simulink model "PMSM_control_model"  (R2024b)
settings: Solver=VariableStepAuto  StartTime=0.0  StopTime=3  RelTol=1e-3
values from neighbouring files (symbols this model uses):
  Is_max = 16    [PMSM_control.m]
  Ls = 5.5e-3    (= 0.0055)    [PMSM_control.m]
  Lsd = 5.5e-3    (= 0.0055)    [PMSM_control.m]
  p = 2    [PMSM_control.m]
  psi_f = 75e-3    (= 0.075)    [PMSM_control.m]
  Us_max = 60    [PMSM_control.m]
libraries: mcbcontrolslib x5, simulink x2
settings Model: Creator=chinm  LastModifiedBy=chinm

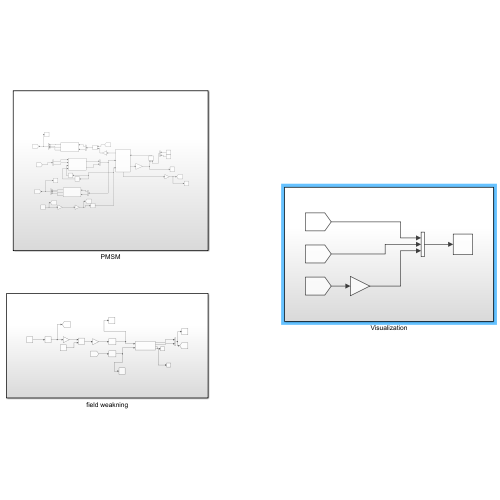
[thumbnail: Simulink's stored preview of the top-level diagram]
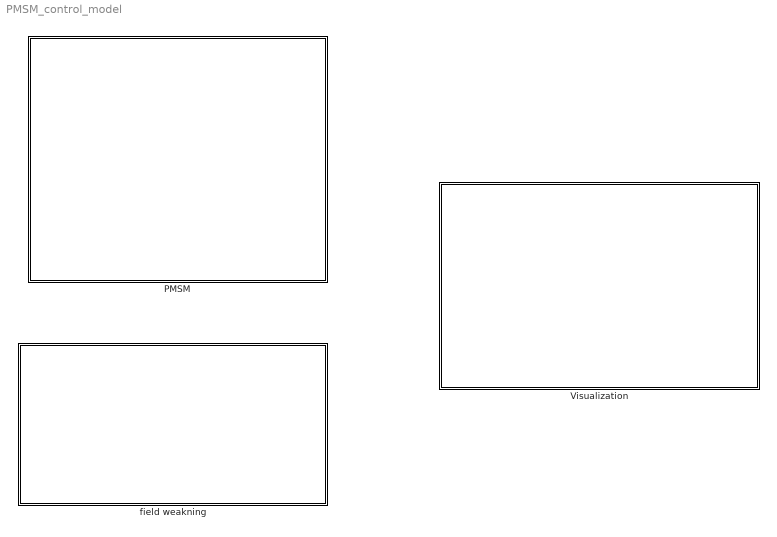
== system PMSM_control_model ==
  PMSM : Subsystem
  Visualization : Subsystem
  field weakning : Subsystem

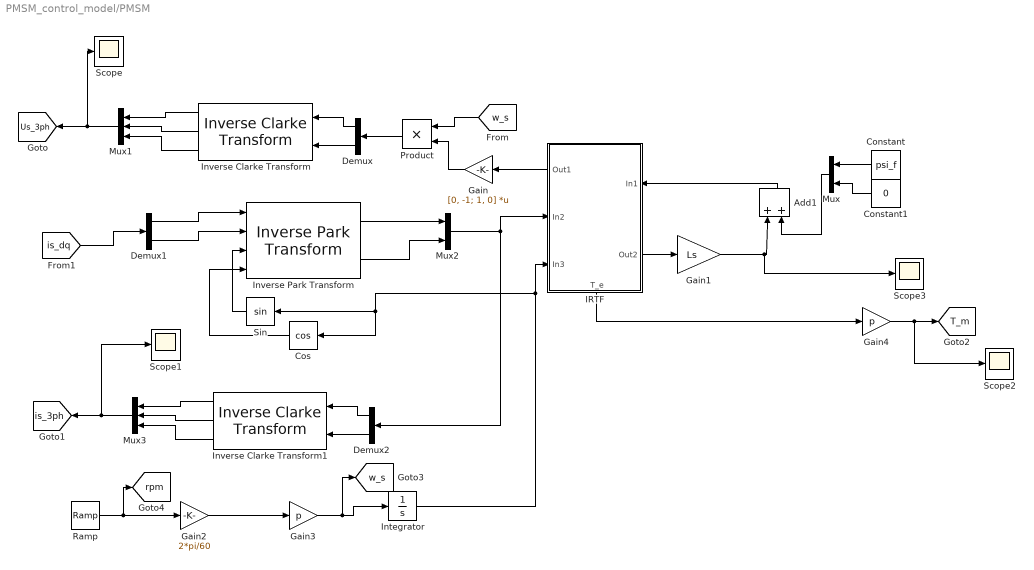
== system PMSM_control_model/PMSM ==
  Add1 : Sum
  Constant : Constant  Value=psi_f
  Constant1 : Constant  Value=0
  Cos : Trigonometry  Operator=cos
  Demux : Demux  Outputs=2
  Demux1 : Demux  Outputs=2
  Demux2 : Demux  Outputs=2
  Gain : Gain  Gain=[0, -1; 1, 0]  Multiplication=Matrix(K*u)
  Gain1 : Gain  Gain=Ls
  Gain2 : Gain  Gain=2*pi/60
  Gain3 : Gain  Gain=p
  Gain4 : Gain  Gain=p
  IRTF : Subsystem
      settings: PortSchema="{\"entries\":[{\"content\":{\"sides\":[{\"content\":{\"connectorIds\":[\"Out3\",\"In1\",\"In2\"]},\"type\":\"ConnectorPlacement.EquallySpacedRectSide\",\"uuid\":\"b4986fb2-c57d-4b73-a735-292653fff6d9\"},{\"content\":{\"connectorIds\":[\"In3\",\"Out1\"],\"side\":\"RIGHT\"},\"type\":\"ConnectorPlacement.EquallySpacedRectSide\",\"uuid\":\"9d0dc8a9-3fda-4760-870c-c4cad97d429b\"},{\"content\":{\"side\":\"TOP\"},\"type\":\"ConnectorPlacement.EquallySpacedRectSide\",\"uuid\":\"e1f646a3-730d-45a9-a867-cd53dcd150be\"},{\"content\":{\"connectorIds\":[\"Out2\"],\"side\":\"BOTTOM\"},\"type\":\"ConnectorPlacement.EquallySpacedRectSide\",\"uuid\":\"c6f4b204-5ea6-4623-acea-3e4f968e6d8a\"}]},\"type\":\"ConnectorPlacement.EquallySpacedConnector\",\"uuid\":\"ab7f54df-393a-4b01-99b4-3432e63bf963\"}],\"packageUris\":[\"http://schema.mathworks.com/mf0/Connector/R2020b\"],\"version\":\"1.0\"}"
  Integrator : Integrator
  Inverse Clarke Transform : mcbcontrolslib/Inverse Clarke Transform  PhaseInput=Two inputs  EnPowerInv=off
      settings: LibrarySourceBlock=mcblib/Controls/Math Transforms/Inverse Clarke Transform
  Inverse Clarke Transform1 : mcbcontrolslib/Inverse Clarke Transform  PhaseInput=Two inputs  EnPowerInv=off
      settings: LibrarySourceBlock=mcblib/Controls/Math Transforms/Inverse Clarke Transform
  Inverse Park Transform : mcbcontrolslib/Inverse Park Transform  PhaseInput=Two inputs  AxisAlignment=D-axis  ThetaInput=Sine and Cosine electrical position  AngleInput=Per-unit  N_points=1024
      settings: LibrarySourceBlock=mcbhdllib/Controls/Math Transforms/Inverse Park Transform
  Mux : Mux  Inputs=2
  Mux1 : Mux  Inputs=3
  Mux2 : Mux  Inputs=2
  Mux3 : Mux  Inputs=3
  Product : Product
  Ramp : simulink/Sources/Ramp  slope=5000  start=0  InitialOutput=0
  Scope{,1..3} (4 alike) : Scope
  Sin : Trigonometry
  tag scope: T_m=global, Us_3ph=global, is_3ph=global, rpm=global, w_s=global
  wires:
  Constant/1 -> Mux/1
  Constant1/1 -> Mux/2
  Mux/1 -> Add1/2
  Integrator/1 -> IRTF/2(In3), Cos/1, Sin/1
  IRTF/2(T_e) -> Gain4/1
  IRTF/1(Out2) -> Gain1/1
  Gain1/1 -> Scope3/1, Add1/1
  Add1/1 -> IRTF/3(In1)
  IRTF/3(Out1) -> Gain/1
  Gain/1 -> Product/2
  [w_s] -> Product/1
  Product/1 -> Demux/1
  Demux/1 -> Inverse Clarke Transform/1
  Demux/2 -> Inverse Clarke Transform/2
  Mux1/1 -> Scope/1, [Us_3ph]
  Inverse Clarke Transform/1 -> Mux1/1
  Inverse Clarke Transform/2 -> Mux1/2
  Inverse Clarke Transform/3 -> Mux1/3
  Inverse Park Transform/1 -> Mux2/1
  Inverse Park Transform/2 -> Mux2/2
  Sin/1 -> Inverse Park Transform/3
  Cos/1 -> Inverse Park Transform/4
  Demux1/1 -> Inverse Park Transform/1
  Demux1/2 -> Inverse Park Transform/2
  [is_dq] -> Demux1/1
  Demux2/2 -> Inverse Clarke Transform1/2
  Inverse Clarke Transform1/3 -> Mux3/3
  Inverse Clarke Transform1/2 -> Mux3/2
  Inverse Clarke Transform1/1 -> Mux3/1
  Mux2/1 -> IRTF/1(In2), Demux2/1
  Mux3/1 -> Scope1/1, [is_3ph]
  Demux2/1 -> Inverse Clarke Transform1/1
  Gain2/1 -> Gain3/1
  Gain3/1 -> [w_s], Integrator/1
  Gain4/1 -> Scope2/1, [T_m]
  Ramp/1 -> [rpm], Gain2/1

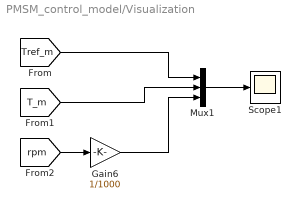
== system PMSM_control_model/Visualization ==
  Gain6 : Gain  Gain=1/1000
  Mux1 : Mux  Inputs=3
  Scope1 : Scope
  wires:
  Mux1/1 -> Scope1/1
  [T_m] -> Mux1/2
  [rpm] -> Gain6/1
  Gain6/1 -> Mux1/3
  [Tref_m] -> Mux1/1

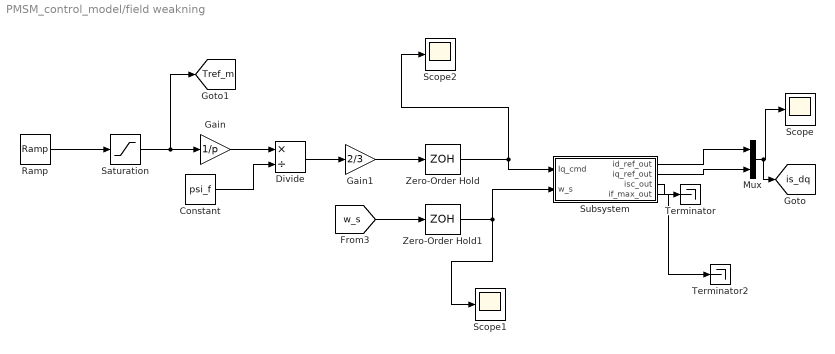
== system PMSM_control_model/field weakning ==
  Constant : Constant  Value=psi_f
  Divide : Product  Inputs=*/
  Gain : Gain  Gain=1/p
  Gain1 : Gain  Gain=2/3
  Mux : Mux  Inputs=2
  Ramp : simulink/Sources/Ramp  slope=10  start=0  InitialOutput=0
  Saturation : Saturate  UpperLimit=2  LowerLimit=0
  Scope : Scope
  Scope1 : Scope
  Scope2 : Scope
  Subsystem : Subsystem
  Terminator : Terminator
  Terminator2 : Terminator
  Zero-Order Hold : ZeroOrderHold  SampleTime=1e-4
  Zero-Order Hold1 : ZeroOrderHold  SampleTime=1e-4
  tag scope: Tref_m=global, is_dq=global
  wires:
  Zero-Order Hold1/1 -> Scope1/1, Subsystem/2(w_s)
  Constant/1 -> Divide/2
  Saturation/1 -> [Tref_m], Gain/1
  Mux/1 -> [is_dq], Scope/1
  Gain/1 -> Divide/1
  [w_s] -> Zero-Order Hold1/1
  Gain1/1 -> Zero-Order Hold/1
  Zero-Order Hold/1 -> Scope2/1, Subsystem/1(Iq_cmd)
  Divide/1 -> Gain1/1
  Subsystem/1(id_ref_out) -> Mux/1
  Subsystem/2(iq_ref_out) -> Mux/2
  Subsystem/3(isc_out) -> Terminator/1
  Subsystem/4(if_max_out) -> Terminator2/1
  Ramp/1 -> Saturation/1

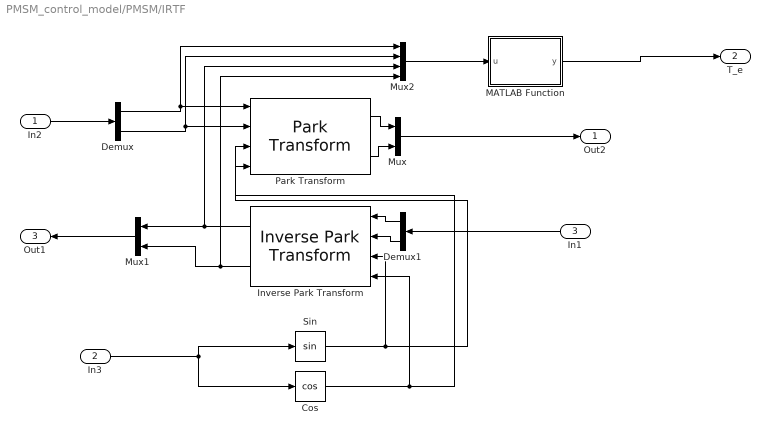
== system PMSM_control_model/PMSM/IRTF ==
  In2 : Inport
  In3 : Inport  Port=2
  In1 : Inport  Port=3
  Cos : Trigonometry  Operator=cos
  Demux : Demux  Outputs=2
  Demux1 : Demux  Outputs=2
  Inverse Park Transform : mcbcontrolslib/Inverse Park Transform  PhaseInput=Two inputs  AxisAlignment=D-axis  ThetaInput=Sine and Cosine electrical position  AngleInput=Per-unit  N_points=1024
  MATLAB Function : MATLAB Function  TreatAsAtomicUnit=on
  Mux : Mux  Inputs=2
  Mux1 : Mux  Inputs=2
  Mux2 : Mux
  Park Transform : mcbcontrolslib/Park Transform  PhaseInput=Two inputs  AxisAlignment=D-axis  ThetaInput=Sine and Cosine electrical position  AngleInput=Per-unit  N_points=1024
  Sin : Trigonometry
  Out2 : Outport
  T_e : Outport  Port=2
  Out1 : Outport  Port=3
  wires:
  Demux/1 -> Mux2/1, Park Transform/1
  Demux/2 -> Mux2/2, Park Transform/2
  Park Transform/1 -> Mux/1
  Park Transform/2 -> Mux/2
  Demux1/1 -> Inverse Park Transform/1
  Demux1/2 -> Inverse Park Transform/2
  Inverse Park Transform/1 -> Mux2/3, Mux1/1
  Inverse Park Transform/2 -> Mux2/4, Mux1/2
  In3/1 -> Sin/1, Cos/1
  Sin/1 -> Park Transform/3, Inverse Park Transform/3
  Cos/1 -> Park Transform/4, Inverse Park Transform/4
  Mux2/1 -> MATLAB Function/1(u)
  MATLAB Function/1(y) -> T_e/1
  In1/1 -> Demux1/1
  Mux1/1 -> Out1/1
  In2/1 -> Demux/1
  Mux/1 -> Out2/1

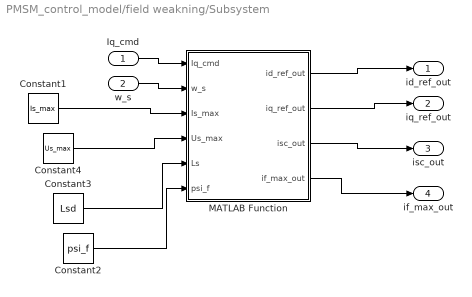
== system PMSM_control_model/field weakning/Subsystem ==
  Iq_cmd : Inport
  w_s : Inport  Port=2
  Constant1 : Constant  Value=Is_max
  Constant2 : Constant  Value=psi_f
  Constant3 : Constant  Value=Lsd
  Constant4 : Constant  Value=Us_max
  MATLAB Function : MATLAB Function  TreatAsAtomicUnit=on
  id_ref_out : Outport
  iq_ref_out : Outport  Port=2
  isc_out : Outport  Port=3
  if_max_out : Outport  Port=4
  wires:
  MATLAB Function/1(id_ref_out) -> id_ref_out/1
  MATLAB Function/2(iq_ref_out) -> iq_ref_out/1
  MATLAB Function/3(isc_out) -> isc_out/1
  MATLAB Function/4(if_max_out) -> if_max_out/1
  Iq_cmd/1 -> MATLAB Function/1(Iq_cmd)
  w_s/1 -> MATLAB Function/2(w_s)
  Constant1/1 -> MATLAB Function/3(Is_max)
  Constant2/1 -> MATLAB Function/6(psi_f)
  Constant3/1 -> MATLAB Function/5(Ls)
  Constant4/1 -> MATLAB Function/4(Us_max)

== matlab function PMSM_control_model/field weakning/Subsystem/MATLAB Function ==
  data: Iq_cmd input; id_ref_out output; w_s input; Is_max input; Us_max input; Ls input; psi_f input; iq_ref_out output; isc_out output; if_max_out output
function [id_ref_out, iq_ref_out, isc_out, if_max_out] = control_logic(Iq_cmd, w_s, Is_max, Us_max, Ls, psi_f)
    % Avoid division by zero
    w_s = max(abs(w_s), 1e-3);
    current = abs(Iq_cmd);

    % Limit current to Is_max
    if current > Is_max
        current = Is_max;
    end

    % Base quantities
    iflm = Us_max / (w_s * Ls);  % voltage ellipse radius
    isc = psi_f / Ls;            % short-circuit current

    % Intersection of voltage ellipse with iq-axis (id = 0)
    iflmq = 0;
    if isc < iflm
        iflmq = sqrt(iflm^2 - isc^2);
    end

    % === Case 1: MTPA ===
    id_ref_MTPA = 0;
    iq_ref_MTPA = current;

    % === Case 2: Field Weakening ===
    iq_ref_FW = current;
    if iflm < current
        iq_ref_FW = iflm;
    end
    temp_fw = max(0, iflm^2 - iq_ref_FW^2);
    id_ref_FW = sqrt(temp_fw) - isc;

    % === Case 3: Maximum Acceleration (MA) ===
    id_ref_MA = (iflm^2 - Is_max^2 - isc^2) / (2 * isc);
    iq_ref_MA = sqrt(max(0, Is_max^2 - id_ref_MA^2));

    % === Default: MTPA ===
    id_ref = id_ref_MTPA;
    iq_ref = iq_ref_MTPA;

    % === FW Mode Trigger ===
    if iq_ref_MTPA > iflmq
        id_ref = id_ref_FW;
        iq_ref = iq_ref_FW;
    end

    % === MA Mode Trigger ===
    if (id_ref^2 + iq_ref^2) > Is_max^2
        id_ref = id_ref_MA;
        iq_ref = iq_ref_MA;
    end

    % === Final Outputs ===
    id_ref_out = id_ref;
    iq_ref_out = iq_ref;
    isc_out = isc;
    if_max_out = iflm;
end

== matlab function PMSM_control_model/PMSM/IRTF/MATLAB Function ==
  data: u input; y output
function y = fcn(u)

y = (u(3)*u(2)-u(4)*u(1))*3/2;
